simulink model "modeSelector"  (R2023a)
settings: Solver=VariableStepAuto  StartTime=0.0  StopTime=10.0  RelTol=1e-3
settings Model: Creator=hugobuurmeijer  LastModifiedBy=hugobuurmeijer

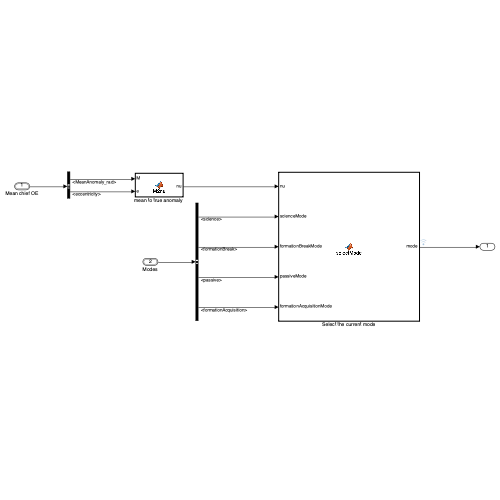
[thumbnail: Simulink's stored preview of the top-level diagram]
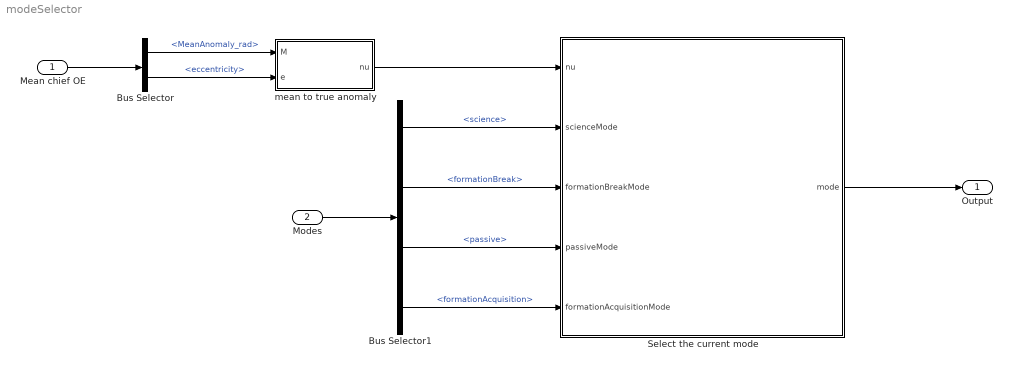
== system modeSelector ==
  Mean chief OE : Inport  OutDataTypeStr=Bus: meanOrbitElements
  Modes : Inport  Port=2  OutDataTypeStr=Bus: modes
  Bus Selector : BusSelector  OutputSignals=MeanAnomaly_rad,eccentricity
  Bus Selector1 : BusSelector  OutputSignals=science,formationBreak,passive,formationAcquisition
  Select the current mode : MATLAB Function  TreatAsAtomicUnit=on
  "mean to true anomaly " : MATLAB Function  TreatAsAtomicUnit=on
  Output : Outport  OutDataTypeStr=string
  wires:
  "mean to true anomaly "/1(nu) -> Select the current mode/1(nu)
  Bus Selector/2 -> "mean to true anomaly "/2(e)  "<eccentricity>"
  Mean chief OE/1 -> Bus Selector/1
  Bus Selector/1 -> "mean to true anomaly "/1(M)  "<MeanAnomaly_rad>"
  Modes/1 -> Bus Selector1/1
  Bus Selector1/1 -> Select the current mode/2(scienceMode)  "<science>"
  Bus Selector1/2 -> Select the current mode/3(formationBreakMode)  "<formationBreak>"
  Bus Selector1/3 -> Select the current mode/4(passiveMode)  "<passive>"
  Bus Selector1/4 -> Select the current mode/5(formationAcquisitionMode)  "<formationAcquisition>"
  Select the current mode/1(mode) -> Output/1

== matlab function modeSelector/Select the current mode ==
  data: nu input; mode output; scienceMode input; formationBreakMode input; passiveMode input; formationAcquisitionMode input
function mode = selectMode(nu, scienceMode, formationBreakMode, passiveMode, formationAcquisitionMode)

mode = selectMode(nu, scienceMode, formationBreakMode, passiveMode, formationAcquisitionMode);

end

== matlab function modeSelector/mean to true anomaly  ==
  data: M input; nu output; e input
function nu = M2nu(M, e)

nu = M2nu(M, e);

end
